simulink model "simu_22a"  (R2022a)
settings: Solver=VariableStepAuto  StartTime=0.0  StopTime=3  RelTol=1e-3
libraries: slpidlib x1
settings Model: Creator=psp_dada  LastModifiedBy=psp_dada
settings ModelReferenceCC: EnableRefExpFcnMdlSchedulingChecks=off
settings RTWCC: Description=Generic Real-Time Target  GPUComputeCapability=5.0
settings ConfigComp: CovBoundaryAbsTol=1.0e-5

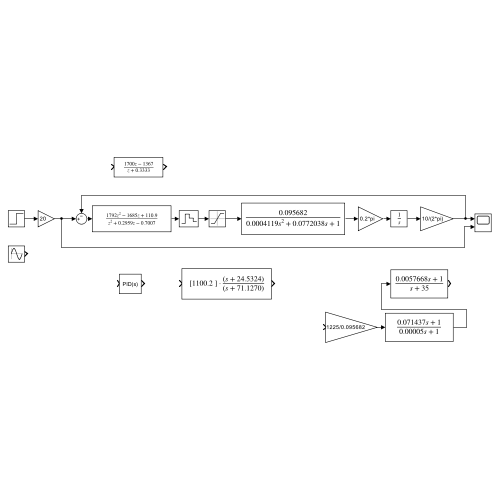
[thumbnail: Simulink's stored preview of the top-level diagram]
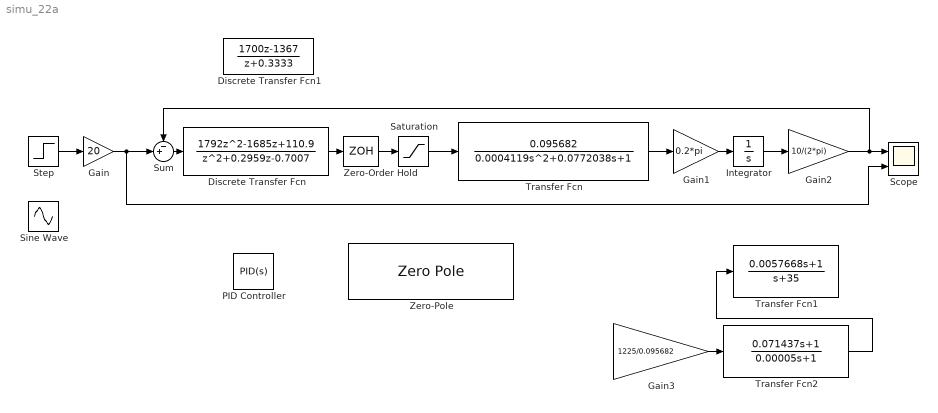
== system simu_22a ==
  Discrete Transfer Fcn : DiscreteTransferFcn  Numerator=[1792 -1685 110.9]  Denominator=[1 0.2959 -0.7007]
  Discrete Transfer Fcn1 : DiscreteTransferFcn  Numerator=[1700 -1367]  Denominator=[1 0.3333]
  Gain : Gain  Gain=20
  Gain1 : Gain  Gain=0.2*pi
  Gain2 : Gain  Gain=10/(2*pi)
  Gain3 : Gain  Gain=1225/0.095682
  Integrator : Integrator
  PID Controller : slpidlib/PID Controller  Controller=PID  Form=Parallel  TimeDomain=Continuous-time  UseExternalTs=off  SampleTime=-1  IntegratorMethod=Forward Euler  FilterMethod=Forward Euler  ControllerParametersSource=internal  P=600  I=0  UseKiTs=off  D=20  N=100  UseFilter=on  TunerSelectOption=Transfer Function Based (PID Tuner App)  InitialConditionSource=internal  InitialConditionForIntegrator=0  InitialConditionForFilter=0  DifferentiatorICPrevScaledInput=0  ExternalReset=none  TrackingMode=off  Kt=1  LimitOutput=off  SatLimitsSource=internal  UpperSaturationLimit=inf  LowerSaturationLimit=-inf  LinearizeAsGain=on  AntiWindupMode=none  Kb=1  POutMin=[]  POutMax=[]  IOutMin=[]  IOutMax=[]  DOutMin=[]  DOutMax=[]  NOutMin=[]  NOutMax=[]  SumOutMin=[]  SumOutMax=[]  SaturationOutMin=[]  SaturationOutMax=[]  PParamMin=[]  PParamMax=[]  IParamMin=[]  IParamMax=[]  DParamMin=[]  DParamMax=[]  NParamMin=[]  NParamMax=[]  KbParamMin=[]  KbParamMax=[]  KtParamMin=[]  KtParamMax=[]  KbOutMin=[]  KbOutMax=[]  KtOutMin=[]  KtOutMax=[]  IntegratorOutMin=[]  IntegratorOutMax=[]  FilterOutMin=[]  FilterOutMax=[]  SumI1OutMin=[]  SumI1OutMax=[]  SumI2OutMin=[]  SumI2OutMax=[]  SumI3OutMin=[]  SumI3OutMax=[]  SumI4OutMin=[]  SumI4OutMax=[]  SumDOutMin=[]  SumDOutMax=[]  DifferentiatorOutMin=[]  DifferentiatorOutMax=[]  FilterDiffOutCoefMin=[]  FilterDiffOutCoefMax=[]  ReciprocalOutMin=[]  ReciprocalOutMax=[]  SumDenOutMin=[]  SumDenOutMax=[]  SumNumOutMin=[]  SumNumOutMax=[]  DivideOutMin=[]  DivideOutMax=[]  UdiffTsProdOutMin=[]  UdiffTsProdOutMax=[]  NTsProdOutMin=[]  NTsProdOutMax=[]  UintegralTsProdOutMin=[]  UintegralTsProdOutMax=[]  UngainTsProdOutMin=[]  UngainTsProdOutMax=[]  IntegratorContinuousStateAttributes=''  IntegratorStateMustResolveToSignalObject=off  IntegratorRTWStateStorageClass=Auto  FilterContinuousStateAttributes=''  FilterStateMustResolveToSignalObject=off  FilterRTWStateStorageClass=Auto  ParallelPVariant=InternalParameters  IdealPVariant=Disabled  IVariant=InternalParameters  DVariant=InternalParameters  IntegratorVariant=Continuous  SatVariant=Disabled  AWVariant=Passthrough  PCopyVariant=Disabled  TRVariant=Disabled  FdbkBlocksVariant=Forward  IdealPFdbkVariant=Disabled  SatFdbkVariant=Disabled  DerivativeFilterVariant=ContFilter  NVariant=InternalParameters  NCopyVariant=Disabled  FilterICVariant=InternalICsFilter  IntegratorICVariant=InternalICs  ExternalResetVariant=Disabled  TRSumVariant=Passthrough  SumFdbkVariant=Disabled  SumVariant=Sum_PID  TsampFilterVariant=InternalTs  TsampNgainVariant=Passthrough  TsampIntegralVariant=Disabled_SignalSpec  ExternalSaturationOutDataTypeStr=Inherit: Same as second input
  Saturation : Saturate  UpperLimit=10000  LowerLimit=-10000
  Scope : Scope  NumInputPorts=2
  Sine Wave : Sin  Frequency=2*pi  SampleTime=0
  Step : Step  Time=0.2  SampleTime=0
  Sum : Sum  Inputs=-+|
  Transfer Fcn : TransferFcn  Numerator=[0.095682]  Denominator=[0.0004119 0.0772038 1]
  Transfer Fcn1 : TransferFcn  Numerator=[0.0057668 1]  Denominator=[1 35]
  Transfer Fcn2 : TransferFcn  Numerator=[0.071437 1]  Denominator=[0.00005 1]
  Zero-Order Hold : ZeroOrderHold  SampleTime=0.01
  Zero-Pole : ZeroPole  Zeros=[-24.5324]  Poles=[-71.1270]  Gain=[1100.2]
  wires:
  Step/1 -> Gain/1
  Gain/1 -> Scope/2, Sum/2
  Sum/1 -> Discrete Transfer Fcn/1
  Saturation/1 -> Transfer Fcn/1
  Transfer Fcn/1 -> Gain1/1
  Gain1/1 -> Integrator/1
  Integrator/1 -> Gain2/1
  Gain2/1 -> Scope/1, Sum/1
  Transfer Fcn2/1 -> Transfer Fcn1/1
  Gain3/1 -> Transfer Fcn2/1
  Zero-Order Hold/1 -> Saturation/1
  Discrete Transfer Fcn/1 -> Zero-Order Hold/1
